simulink model "masterFile"  (R2016b)
settings: Solver=VariableStepAuto  StartTime=0.0  StopTime=inf  RelTol=1e-3
settings Model: Creator=Borja Martos  LastModifiedBy=Borja Martos

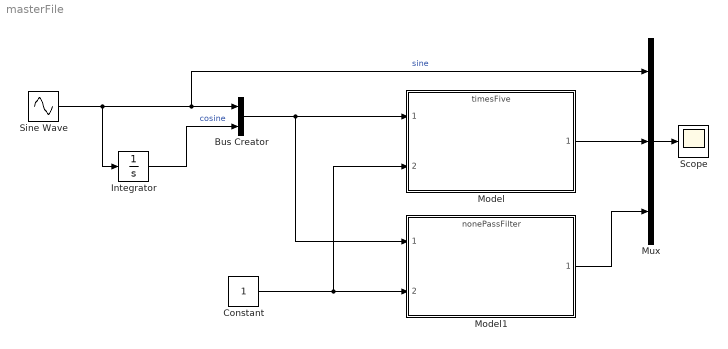
== system masterFile ==
  Bus Creator : BusCreator  Inputs=2
  Constant : Constant
  Integrator : Integrator
  Model : ModelReference  ModelNameDialog=timesFive.slx  SimulationMode=Normal  ModelReferenceVersion=1.7
  Model1 : ModelReference  ModelNameDialog=nonePassFilter.slx  SimulationMode=Normal  ModelReferenceVersion=1.9
  Mux : Mux  Inputs=3
  Scope : Scope
  Sine Wave : Sin  SampleTime=0
  wires:
  Model/1 -> Mux/2
  Mux/1 -> Scope/1
  Constant/1 -> Model1/2, Model/2
  Sine Wave/1 -> Integrator/1, Mux/1, Bus Creator/1  "sine"
  Integrator/1 -> Bus Creator/2  "cosine"
  Bus Creator/1 -> Model1/1, Model/1
  Model1/1 -> Mux/3
